simulink model "exemplo_bloco_controle_PID"  (R2019a)
settings: Solver=ode45  StartTime=0.0  StopTime=200.0  RelTol=1e-3  EnableMultiTasking=on
settings Model: Creator=Mauricio  LastModifiedBy=YecidMoreno
settings DataIOCC: LimitDataPoints=on  SaveFormat=Array  ReturnWorkspaceOutputs=off
settings OptimizationCC: InitFltsAndDblsToZero=on  LifeSpan=inf
settings DebuggingCC: SaveWithParameterizedLinksMsg=none  SignalResolutionControl=TryResolveAllWithWarning  SolverPrmCheckMsg=warning  MultiTaskDSMMsg=warning  MultiTaskCondExecSysMsg=none  FcnCallInpInsideContextMsg=warning  SFUnexpectedBacktrackingDiag=warning  SFNoUnconditionalDefaultTransitionDiag=warning  SFExecutionAtInitializationDiag=none  ArithmeticOperatorsInVariantConditions=warning
settings HardwareCC: ProdBitPerPointer=32  ProdBitPerSizeT=32  ProdBitPerPtrDiffT=32  ProdLargestAtomicFloat=None  ProdIntDivRoundTo=Undefined  ProdEndianess=Unspecified  ProdWordSize=32  ProdHWDeviceType=32-bit Generic
settings ModelReferenceCC: PropagateSignalLabelsOutOfModel=off
settings SFSimCC: SimUseLocalCustomCode=off
settings RTWCC: RTWUseLocalCustomCode=off
settings CodeAppCC: StateflowObjectComments=on
settings GRTTargetCC: TargetFcnLib=ansi_tfl_tmw.mat  TargetLangStandard=C89/C90 (ANSI)  GeneratePreprocessorConditionals=Disable all  CombineOutputUpdateFcns=off  GRTInterface=on
settings ConfigComp: CovMetricSettings=dw  CovHtmlReporting=on  CovSaveCumulativeToWorkspaceVar=on  CovSaveSingleToWorkspaceVar=on  CovExternalEMLEnable=off  CovSFcnEnable=off

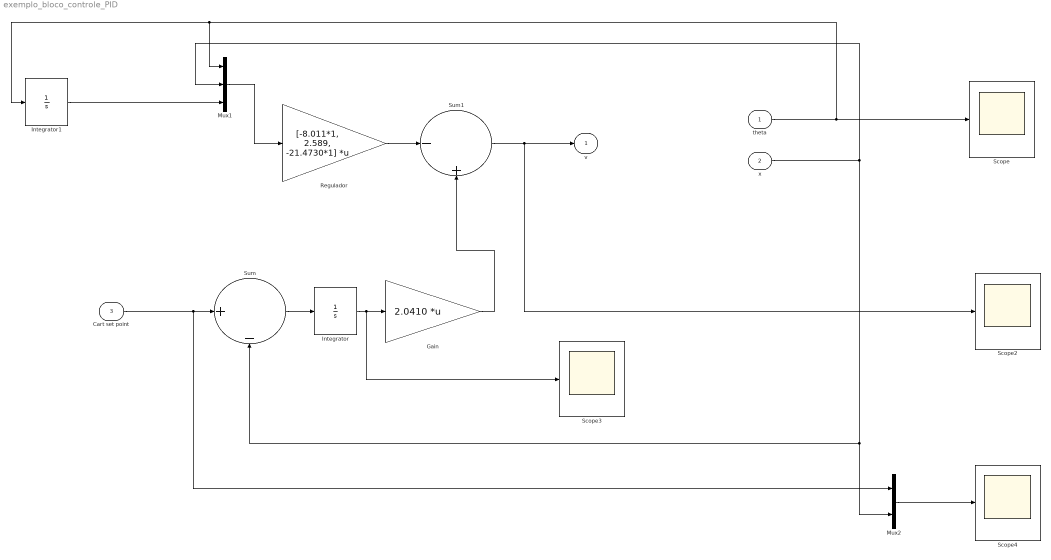
== system exemplo_bloco_controle_PID ==
  theta : Inport
  x : Inport  Port=2
  Cart set point : Inport  Port=3
  Gain : Gain  Gain=2.0410  Multiplication=Matrix(K*u)
  Integrator : Integrator
  Integrator1 : Integrator
  Mux1 : Mux  Inputs=3
  Mux2 : Mux  Inputs=2
  Regulador : Gain  Gain=[-8.011*1, 2.589, -21.4730*1]  Multiplication=Matrix(K*u)
  Scope{,2..4} (4 alike) : Scope
  Sum : Sum  Inputs=|+-
  Sum1 : Sum  Inputs=|-+
  v : Outport
  wires:
  Regulador/1 -> Sum1/1
  Cart set point/1 -> Mux2/1, Sum/1
  Mux2/1 -> Scope4/1
  Gain/1 -> Sum1/2
  Sum1/1 -> v/1, Scope2/1
  Integrator/1 -> Scope3/1, Gain/1
  theta/1 -> Mux1/1, Integrator1/1, Scope/1
  Integrator1/1 -> Mux1/3
  Sum/1 -> Integrator/1
  x/1 -> Mux2/2, Sum/2, Mux1/2
  Mux1/1 -> Regulador/1
